simulink model "ModelEnv"  (R2020b)
settings: Solver=VariableStepAuto  StartTime=0.0  StopTime=Tf  RelTol=1e-3
undefined symbols (not defined in the file): c, M, mdot, R
libraries: dspsrcs4 x2, rllib x1
settings Model: Creator=masdoua1  LastModifiedBy=masdoua1

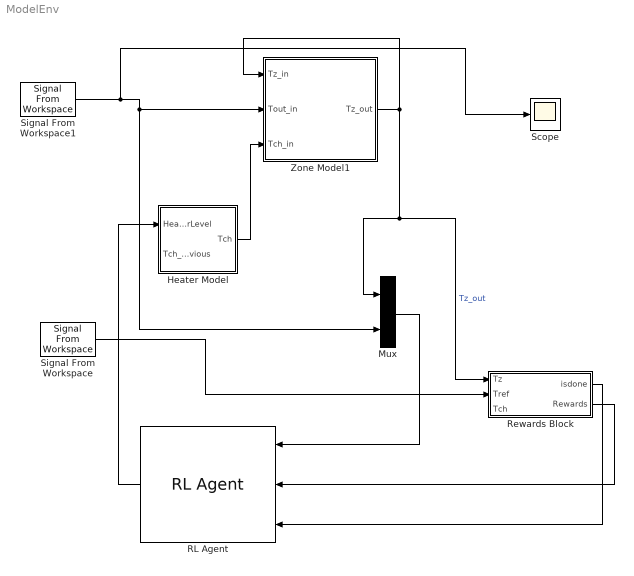
== system ModelEnv ==
  Heater Model : Subsystem
  Mux : Mux  Inputs=2
  RL Agent : rllib/RL Agent  Agent=agent  ProvideReward=on  ProvideIsDone=on  ProvideCumRwd=off  TreatAsDirectFeedthrough=on  CollectLoggedSignals=on  CollectModelStates=on
  Rewards Block : Subsystem
  Scope : Scope
  Signal From Workspace : dspsrcs4/Signal From Workspace  X=Tref  Ts=1  nsamps=1  OutputAfterFinalValue=Setting to zero  ignoreOrWarnInputAndFrameLengths=off  OutputFrames=off
  Signal From Workspace1 : dspsrcs4/Signal From Workspace  X=Tout  Ts=1  nsamps=1  OutputAfterFinalValue=Setting to zero  ignoreOrWarnInputAndFrameLengths=off  OutputFrames=off
  Zone Model1 : Subsystem
  wires:
  Signal From Workspace/1 -> Rewards Block/2(Tref)
  Rewards Block/2(Rewards) -> RL Agent/2
  Rewards Block/1(isdone) -> RL Agent/3
  RL Agent/1 -> Heater Model/1(HeaterLevel)
  Mux/1 -> RL Agent/1
  Heater Model/1(Tch) -> Zone Model1/3(Tch_in)
  Zone Model1/1(Tz_out) -> Rewards Block/1(Tz), Mux/1, Zone Model1/1(Tz_in)  "Tz_out"
  Signal From Workspace1/1 -> Scope/1, Zone Model1/2(Tout_in), Mux/2

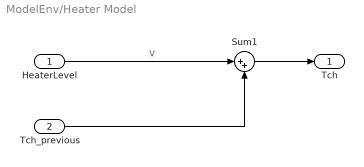
== system ModelEnv/Heater Model ==
  HeaterLevel : Inport
  Tch_previous : Inport  Port=2
  Sum1 : Sum  Inputs=|++
  Tch : Outport
  wires:
  HeaterLevel/1 -> Sum1/1  "V"
  Sum1/1 -> Tch/1
  Tch_previous/1 -> Sum1/2

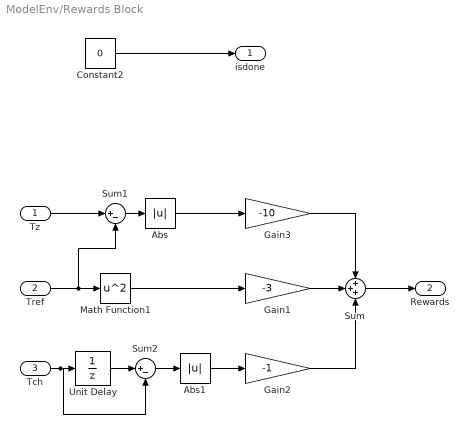
== system ModelEnv/Rewards Block ==
  Tz : Inport
  Tref : Inport  Port=2
  Tch : Inport  Port=3
  Abs : Abs
  Abs1 : Abs
  Constant2 : Constant  Value=0
  Gain1 : Gain  Gain=-3
  Gain2 : Gain  Gain=-1
  Gain3 : Gain  Gain=-10
  Math Function1 : Math  Operator=square  SignedPower=on  SaturateOnIntegerOverflow=on
  Sum : Sum  Inputs=+++
  Sum1 : Sum  Inputs=|+-
  Sum2 : Sum  Inputs=|+-
  Unit Delay : UnitDelay  SampleTime=-1  HasFrameUpgradeWarning=on
  isdone : Outport  VectorParamsAs1DForOutWhenUnconnected=off
  Rewards : Outport  Port=2  VectorParamsAs1DForOutWhenUnconnected=off
  wires:
  Constant2/1 -> isdone/1
  Tz/1 -> Sum1/1
  Tref/1 -> Sum1/2, Math Function1/1
  Tch/1 -> Sum2/2, Unit Delay/1
  Sum/1 -> Rewards/1
  Math Function1/1 -> Gain1/1
  Sum2/1 -> Abs1/1
  Gain2/1 -> Sum/3
  Gain1/1 -> Sum/2
  Gain3/1 -> Sum/1
  Unit Delay/1 -> Sum2/1
  Sum1/1 -> Abs/1
  Abs/1 -> Gain3/1
  Abs1/1 -> Gain2/1

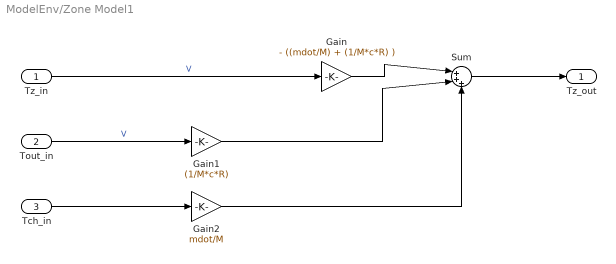
== system ModelEnv/Zone Model1 ==
  Tz_in : Inport
  Tout_in : Inport  Port=2
  Tch_in : Inport  Port=3
  Gain : Gain  Gain=- ((mdot/M) + (1/M*c*R) )
  Gain1 : Gain  Gain=(1/M*c*R)
  Gain2 : Gain  Gain=mdot/M
  Sum : Sum  Inputs=|+++
  Tz_out : Outport  VectorParamsAs1DForOutWhenUnconnected=off
  wires:
  Tz_in/1 -> Gain/1  "V"
  Gain/1 -> Sum/1
  Tout_in/1 -> Gain1/1  "V"
  Gain1/1 -> Sum/2
  Tch_in/1 -> Gain2/1
  Gain2/1 -> Sum/3
  Sum/1 -> Tz_out/1
